simulink model "MHILSimHWImpl"  (R2024a)
settings: Solver=FixedStepDiscrete  StartTime=0.0  StopTime=2e-4  FixedStep=4e-9  RelTol=1e-3
values from neighbouring files (symbols this model uses):
  cfg = tddbl_model    [HILSimModel.m]
undefined symbols (not defined in the file or in its folder): AXI4, dt, hw, ip, Lite, xc7z020clg400
libraries: hdlBasic x1497, hdlUtilities x3, vmcUtilities x1
(part 3 of 11)

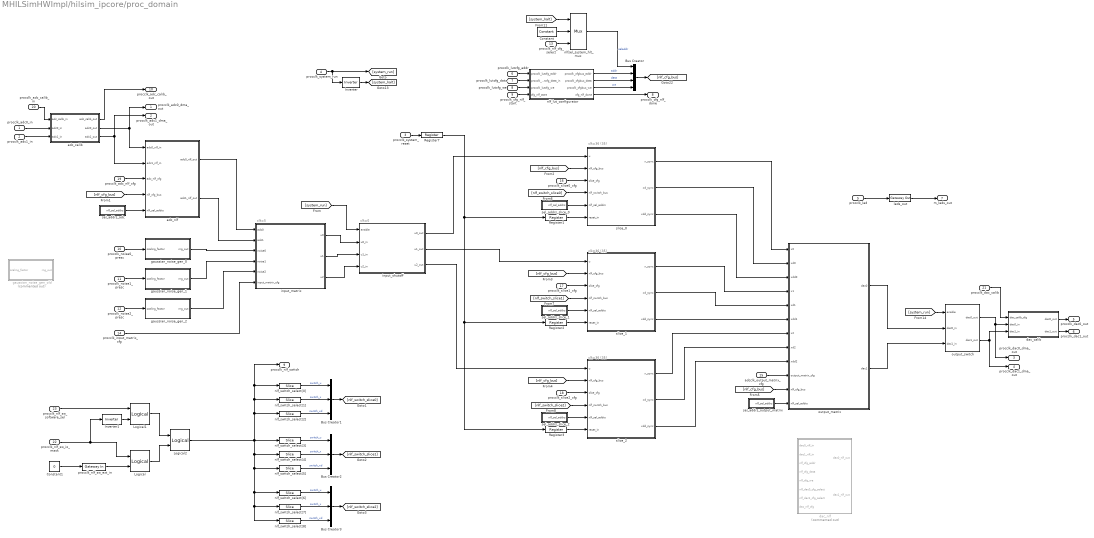
== system MHILSimHWImpl/hilsim_ipcore/proc_domain ==
  note: clk=5
  note: clk=0
  note: clk=36 (35)
  note: clk=36 (35)
  note: clk=36 (35)
  procclk_adc0_in : Inport
  procclk_adc1_in : Inport  Port=2
  procclk_system_reset : Inport  Port=3
  procclk_system_run : Inport  Port=4
  procclk_led : Inport  Port=5
  procclk_lutcfg_addr : Inport  Port=6
  procclk_lutcfg_data : Inport  Port=7
  procclk_lutcfg_we : Inport  Port=8
  procclk_cfg_nlf_start : Inport  Port=9
  procclk_noise0_presc : Inport  Port=10
  procclk_noise1_presc : Inport  Port=11
  procclk_noise2_presc : Inport  Port=12
  procclk_nlf_cfg_select : Inport  Port=13
  procclk_input_matrix_cfg : Inport  Port=14
  adcclk_output_matrix_cfg : Inport  Port=15
  procclk_slice0_cfg : Inport  Port=16
  procclk_slice1_cfg : Inport  Port=17
  procclk_slice2_cfg : Inport  Port=18
  procclk_adc_nlf_cfg : Inport  Port=19
  procclk_adc_calib_in : Inport  Port=20
  procclk_dac_calib : Inport  Port=21
  procclk_nlf_sw_io_mask : Inport  Port=22
  procclk_nlf_sw_software_sel : Inport  Port=23
  Bus Creator : BusCreator  Inputs=4
  Bus Creator1 : BusCreator  Inputs=3
  Bus Creator2 : BusCreator  Inputs=3
  Bus Creator3 : BusCreator  Inputs=3
  Constant : hdlBasic/Constant  const=255  gui_display_data_type=Fixed-point  arith_type=Unsigned  n_bits=8  bin_pt=0  preci_type=Single  exp_width=8  frac_width=24  explicit_period=off  period=1  XmcBlockStatus=1  maskContainerNames=tabcontainer1  block_type=constant  block_config=sysgen:Constant_config
  Constant1 : Constant  Value=0
  Inverter : hdlBasic/Inverter  en=off  latency=0  XmcBlockStatus=1  maskContainerNames=group2  block_type=inv  block_config=sysgen:Inverter_config
  Inverter1 : hdlBasic/Inverter  en=off  latency=0  XmcBlockStatus=1  maskContainerNames=group2  block_type=inv  block_config=sysgen:Inverter_config
  Logical : hdlBasic/Logical  logical_function=AND  inputs=2  en=off  latency=1  precision=Full  arith_type=Unsigned  n_bits=16  bin_pt=0  align_bp=on  overflow=[]  quantization=[]  XmcBlockStatus=1  maskContainerNames=tabcontainer1  block_type=logical  block_config=sysgen:Logical_config
  Logical1 : hdlBasic/Logical  logical_function=AND  inputs=2  en=off  latency=1  precision=Full  arith_type=Unsigned  n_bits=16  bin_pt=0  align_bp=on  overflow=[]  quantization=[]  XmcBlockStatus=1  maskContainerNames=tabcontainer1  block_type=logical  block_config=sysgen:Logical_config
  Logical2 : hdlBasic/Logical  logical_function=OR  inputs=2  en=off  latency=0  precision=Full  arith_type=Unsigned  n_bits=16  bin_pt=0  align_bp=on  overflow=[]  quantization=[]  XmcBlockStatus=1  maskContainerNames=tabcontainer1  block_type=logical  block_config=sysgen:Logical_config
  Register{1..3,7} (4 alike) : hdlBasic/Register  init=0  rst=off  en=off  XmcBlockStatus=1  maskContainerNames=tabcontainer1  block_type=register  block_config=sysgen:Register_config
  adc_calib : Subsystem
  adc_nlf : Subsystem
  dac_calib : Subsystem
  dac_nlf : Subsystem  Commented=on
  gaussian_noise_gen_0 : Subsystem
  gaussian_noise_gen_1 : Subsystem
  gaussian_noise_gen_2 : Subsystem
  gaussian_noise_gen_old : Subsystem  Commented=on
  input_matrix : Subsystem
  input_shutoff : Subsystem
  leds_out : hdlBasic/Gateway Out  inherit_from_input=off  hdl_port=on  rows=1  columns=1  UseAsDAC=off  DACChannel='1'  interface=None  automatic_assignment=on  address_offset=hex2dec('00')  intf_name=''  intf_description=''  timing_constraint=None  locs_specified=off  LOCs={}  io_standard={}  XmcBlockStatus=1  maskContainerNames=group4  block_type=gatewayout  block_config=sysgen:gateway_out_config  block_width_w=590  block_height_w=620  block_width=620  block_height=750
  nlf_lut_configurator : Subsystem
  nlf_switch_select[0] : hdlBasic/Slice  nbits=0  boolean_output=on  mode=Lower Bit Location + Width  bit1=0  base1=MSB of Input  bit0=0  base0=LSB of Input  XmcBlockStatus=1  maskContainerNames=group1  block_type=slice  block_config=sysgen:Slice_config
  nlf_switch_select[1] : hdlBasic/Slice  nbits=0  boolean_output=on  mode=Lower Bit Location + Width  bit1=0  base1=MSB of Input  bit0=1  base0=LSB of Input  XmcBlockStatus=1  maskContainerNames=group1  block_type=slice  block_config=sysgen:Slice_config
  nlf_switch_select[2] : hdlBasic/Slice  nbits=0  boolean_output=on  mode=Lower Bit Location + Width  bit1=0  base1=MSB of Input  bit0=2  base0=LSB of Input  XmcBlockStatus=1  maskContainerNames=group1  block_type=slice  block_config=sysgen:Slice_config
  nlf_switch_select[3] : hdlBasic/Slice  nbits=0  boolean_output=on  mode=Lower Bit Location + Width  bit1=0  base1=MSB of Input  bit0=3  base0=LSB of Input  XmcBlockStatus=1  maskContainerNames=group1  block_type=slice  block_config=sysgen:Slice_config
  nlf_switch_select[4] : hdlBasic/Slice  nbits=0  boolean_output=on  mode=Lower Bit Location + Width  bit1=0  base1=MSB of Input  bit0=4  base0=LSB of Input  XmcBlockStatus=1  maskContainerNames=group1  block_type=slice  block_config=sysgen:Slice_config
  nlf_switch_select[5] : hdlBasic/Slice  nbits=0  boolean_output=on  mode=Lower Bit Location + Width  bit1=0  base1=MSB of Input  bit0=5  base0=LSB of Input  XmcBlockStatus=1  maskContainerNames=group1  block_type=slice  block_config=sysgen:Slice_config
  nlf_switch_select[6] : hdlBasic/Slice  nbits=0  boolean_output=on  mode=Lower Bit Location + Width  bit1=0  base1=MSB of Input  bit0=6  base0=LSB of Input  XmcBlockStatus=1  maskContainerNames=group1  block_type=slice  block_config=sysgen:Slice_config
  nlf_switch_select[7] : hdlBasic/Slice  nbits=0  boolean_output=on  mode=Lower Bit Location + Width  bit1=0  base1=MSB of Input  bit0=7  base0=LSB of Input  XmcBlockStatus=1  maskContainerNames=group1  block_type=slice  block_config=sysgen:Slice_config
  nlf_switch_select[8] : hdlBasic/Slice  nbits=0  boolean_output=on  mode=Lower Bit Location + Width  bit1=0  base1=MSB of Input  bit0=8  base0=LSB of Input  XmcBlockStatus=1  maskContainerNames=group1  block_type=slice  block_config=sysgen:Slice_config
  nlfsel_system_hlt_mux : hdlBasic/Mux  inputs=2  en=off  latency=1  precision=Full  arith_type=Unsigned  n_bits=16  bin_pt=14  quantization=Truncate  overflow=Wrap  XmcBlockStatus=1  maskContainerNames=tabcontainer1  block_type=mux  block_config=sysgen:Mux_config
  output_matrix : Subsystem
  output_switch : Subsystem
  procclk_nlf_sw_ext_in : hdlBasic/Gateway In  gui_display_data_type=Fixed-point  arith_type=Unsigned  n_bits=9  bin_pt=0  preci_type=Single  exp_width=8  frac_width=24  rows=1  columns=1  quantization="Round  (unbiased: +/- Inf)"  overflow=Saturate  period=1  UseAsADC=off  ADCChannel='1'  interface=None  automatic_assignment=on  address_offset=hex2dec('00')  intf_name=''  intf_description=''  default_value=0  timing_constraint=None  locs_specified=off  LOCs={}  io_standard={}  inherit_from_input=off  hdl_port=on  XmcBlockStatus=1  maskContainerNames=group4  block_type=gatewayin  block_config=sysgen:gateway_in_config  block_width_w=590  block_height_w=620  block_width=640  block_height=850
  sel_addrs_adc : Subsystem
  sel_addrs_output_matrix : Subsystem
  sel_addrs_slice_0 : Subsystem
  sel_addrs_slice_1 : Subsystem
  sel_addrs_slice_2 : Subsystem
  slice_0 : Subsystem
  slice_1 : Subsystem
  slice_2 : Subsystem
  procclk_adc0_dma_out : Outport
  procclk_adc1_dma_out : Outport  Port=2
  procclk_dac0_dma_out : Outport  Port=3
  procclk_dac1_dma_out : Outport  Port=4
  procclk_dac0_out : Outport  Port=5
  procclk_dac1_out : Outport  Port=6
  m_leds_out : Outport  Port=7
  procclk_cfg_nlf_done : Outport  Port=8
  procclk_nlf_switch : Outport  Port=9
  procclk_adc_calib_out : Outport  Port=10
  wires:
  leds_out/1 -> m_leds_out/1
  procclk_led/1 -> leds_out/1
  procclk_lutcfg_addr/1 -> nlf_lut_configurator/1(procclk_lutcfg_addr)
  procclk_lutcfg_we/1 -> nlf_lut_configurator/3(procclk_lutcfg_we)
  procclk_lutcfg_data/1 -> nlf_lut_configurator/2(procclk_lutcfg_data_in)
  procclk_cfg_nlf_start/1 -> nlf_lut_configurator/4(cfg_nlf_start)
  nlf_lut_configurator/4(cfg_nlf_done) -> procclk_cfg_nlf_done/1
  procclk_slice0_cfg/1 -> slice_0/3(slice_cfg)
  gaussian_noise_gen_1/1(rng_out) -> input_matrix/4(noise1)
  gaussian_noise_gen_2/1(rng_out) -> input_matrix/5(noise2)
  procclk_noise0_presc/1 -> gaussian_noise_gen_0/1(scaling_factor)
  procclk_noise2_presc/1 -> gaussian_noise_gen_2/1(scaling_factor)
  procclk_noise1_presc/1 -> gaussian_noise_gen_1/1(scaling_factor)
  procclk_input_matrix_cfg/1 -> input_matrix/6(input_matrix_cfg)
  input_matrix/1(u0) -> input_shutoff/2(u0_in)
  input_matrix/2(u1) -> input_shutoff/3(u1_in)
  input_matrix/3(u2) -> input_shutoff/4(u2_in)
  [system_run] -> input_shutoff/1(enable)
  nlf_lut_configurator/1(procclk_cfgbus_addr) -> Bus Creator/2  "addr"
  nlf_lut_configurator/2(procclk_cfgbus_data) -> Bus Creator/3  "data"
  nlf_lut_configurator/3(procclk_cfgbus_we) -> Bus Creator/4  "we"
  input_shutoff/1(u0_out) -> slice_0/1(u)
  input_shutoff/2(u1_out) -> slice_1/1(u)
  input_shutoff/3(u2_out) -> slice_2/1(u)
  slice_0/1(x_sync) -> output_matrix/1(x0)
  slice_0/2(xd_sync) -> output_matrix/2(xd0)
  slice_1/1(x_sync) -> output_matrix/4(x1)
  slice_1/2(xd_sync) -> output_matrix/5(xd1)
  slice_2/1(x_sync) -> output_matrix/7(x2)
  slice_2/2(xd_sync) -> output_matrix/8(xd2)
  [system_run] -> output_switch/1(enable)
  adcclk_output_matrix_cfg/1 -> output_matrix/10(output_matrix_cfg)
  procclk_system_run/1 -> [system_run], Inverter/1
  Inverter/1 -> [system_halt]
  adc_nlf/2(adc1_nlf_out) -> input_matrix/2(adc1)
  adc_nlf/1(adc0_nlf_out) -> input_matrix/1(adc0)
  procclk_adc_nlf_cfg/1 -> adc_nlf/3(adc_nlf_cfg)
  gaussian_noise_gen_0/1(rng_out) -> input_matrix/3(noise0)
  procclk_system_reset/1 -> Register7/1
  Register7/1 -> Register3/1, Register2/1, Register1/1
  Register1/1 -> slice_0/6(reset_in)
  procclk_adc0_in/1 -> adc_calib/2(adc0_in)
  procclk_adc1_in/1 -> adc_calib/3(adc1_in)
  adc_calib/1(adc_calib_out) -> procclk_adc_calib_out/1
  procclk_adc_calib_in/1 -> adc_calib/1(adc_calib_in)
  adc_calib/2(adc0_out) -> procclk_adc0_dma_out/1, adc_nlf/1(adc0_nlf_in)
  adc_calib/3(adc1_out) -> procclk_adc1_dma_out/1, adc_nlf/2(adc1_nlf_in)
  output_matrix/1(dac0) -> output_switch/2(dac0_in)
  output_matrix/2(dac1) -> output_switch/3(dac1_in)
  dac_calib/1(dac0_out) -> procclk_dac0_out/1
  dac_calib/2(dac1_out) -> procclk_dac1_out/1
  output_switch/1(dac0_out) -> procclk_dac0_dma_out/1, dac_calib/2(dac0_in)
  output_switch/2(dac1_out) -> dac_calib/3(dac1_in), procclk_dac1_dma_out/1
  procclk_dac_calib/1 -> dac_calib/1(dac_calib_cfg)
  slice_0/3(xdd_sync) -> output_matrix/3(xdd0)
  slice_1/3(xdd_sync) -> output_matrix/6(xdd1)
  slice_2/3(xdd_sync) -> output_matrix/9(xdd2)
  Bus Creator/1 -> [nlf_cfg_bus]
  [nlf_cfg_bus] -> slice_0/2(nlf_cfg_bus)
  sel_addrs_slice_0/1(nlf_sel_addrs) -> slice_0/5(nlf_sel_addrs)
  [system_halt] -> nlfsel_system_hlt_mux/1
  nlfsel_system_hlt_mux/1 -> Bus Creator/1  "seladdr"
  procclk_slice1_cfg/1 -> slice_1/3(slice_cfg)
  Register2/1 -> slice_1/6(reset_in)
  sel_addrs_slice_1/1(nlf_sel_addrs) -> slice_1/5(nlf_sel_addrs)
  procclk_slice2_cfg/1 -> slice_2/3(slice_cfg)
  Register3/1 -> slice_2/6(reset_in)
  sel_addrs_slice_2/1(nlf_sel_addrs) -> slice_2/5(nlf_sel_addrs)
  sel_addrs_output_matrix/1(nlf_sel_addrs) -> output_matrix/12(nlf_sel_addrs)
  [nlf_cfg_bus] -> slice_1/2(nlf_cfg_bus)
  [nlf_cfg_bus] -> slice_2/2(nlf_cfg_bus)
  [nlf_cfg_bus] -> output_matrix/11(nlf_cfg_bus)
  sel_addrs_adc/1(nlf_sel_addrs) -> adc_nlf/5(nlf_sel_addrs)
  [nlf_cfg_bus] -> adc_nlf/4(nlf_cfg_bus)
  nlf_switch_select[0]/1 -> Bus Creator1/1  "switch_u"
  nlf_switch_select[1]/1 -> Bus Creator1/2  "switch_x"
  nlf_switch_select[2]/1 -> Bus Creator1/3  "switch_xd"
  Bus Creator1/1 -> [nlf_switch_slice0]
  [nlf_switch_slice0] -> slice_0/4(nlf_switch_bus)
  Bus Creator2/1 -> [nlf_switch_slice1]
  nlf_switch_select[5]/1 -> Bus Creator2/3  "switch_xd"
  nlf_switch_select[3]/1 -> Bus Creator2/1  "switch_u"
  nlf_switch_select[4]/1 -> Bus Creator2/2  "switch_x"
  [nlf_switch_slice1] -> slice_1/4(nlf_switch_bus)
  nlf_switch_select[6]/1 -> Bus Creator3/1  "switch_u"
  nlf_switch_select[8]/1 -> Bus Creator3/3  "switch_xd"
  nlf_switch_select[7]/1 -> Bus Creator3/2  "switch_x"
  Bus Creator3/1 -> [nlf_switch_slice2]
  [nlf_switch_slice2] -> slice_2/4(nlf_switch_bus)
  Logical2/1 -> procclk_nlf_switch/1, nlf_switch_select[0]/1, nlf_switch_select[1]/1, nlf_switch_select[2]/1, nlf_switch_select[8]/1, nlf_switch_select[7]/1, nlf_switch_select[6]/1, nlf_switch_select[5]/1, nlf_switch_select[4]/1, nlf_switch_select[3]/1
  Constant1/1 -> procclk_nlf_sw_ext_in/1
  procclk_nlf_sw_ext_in/1 -> Logical/2
  Inverter1/1 -> Logical1/2
  procclk_nlf_sw_io_mask/1 -> Inverter1/1, Logical/1
  procclk_nlf_sw_software_sel/1 -> Logical1/1
  Logical1/1 -> Logical2/1
  Logical/1 -> Logical2/2
  Constant/1 -> nlfsel_system_hlt_mux/2
  procclk_nlf_cfg_select/1 -> nlfsel_system_hlt_mux/3

== system MHILSimHWImpl/hilsim_ipcore/proc_domain/adc_calib ==
  adc_calib_in : Inport
  adc0_in : Inport  Port=2
  adc1_in : Inport  Port=3
  Bus Creator8 : BusCreator  Inputs=2
  Bus Selector9 : BusSelector  OutputSignals=signal1,signal2,signal3,signal4
  Register{1..3,17} (4 alike) : hdlBasic/Register  init=0  rst=off  en=off  XmcBlockStatus=1  maskContainerNames=tabcontainer1  block_type=register  block_config=sysgen:Register_config
  adc0_calib_add : hdlBasic/AddSub  mode=Addition  use_carryin=off  use_carryout=off  en=off  latency=1  precision=User Defined  arith_type="Signed  (2's comp)"  n_bits=dt.slice.sz  bin_pt=dt.slice.bin  quantization=Truncate  overflow=Wrap  use_behavioral_HDL=off  hw_selection=Fabric  pipelined=off  XmcBlockStatus=1  maskContainerNames=tabcontainer1  block_type=addsub  block_config=sysgen:Addsub_config
  adc0_calib_mul : hdlBasic/Mult  precision=User Defined  arith_type="Signed  (2's comp)"  n_bits=dt.slice.sz  bin_pt=dt.slice.bin  quantization=Truncate  overflow=Wrap  en=off  latency=3  opt_float=off  fp_mult_usage=No Usage  use_behavioral_HDL=off  opt=Speed  use_embedded=on  optimum_pipeline=off  pipeline=on  use_rpm=on  placement_style=Triangular  XmcBlockStatus=1  maskContainerNames=group1  block_type=mult  block_config=sysgen:Mult_config  block_width=598  block_height=876
  adc1_calib_add : hdlBasic/AddSub  mode=Addition  use_carryin=off  use_carryout=off  en=off  latency=1  precision=User Defined  arith_type="Signed  (2's comp)"  n_bits=dt.slice.sz  bin_pt=dt.slice.bin  quantization=Truncate  overflow=Wrap  use_behavioral_HDL=off  hw_selection=Fabric  pipelined=off  XmcBlockStatus=1  maskContainerNames=tabcontainer1  block_type=addsub  block_config=sysgen:Addsub_config
  adc1_calib_mul : hdlBasic/Mult  precision=User Defined  arith_type="Signed  (2's comp)"  n_bits=dt.slice.sz  bin_pt=dt.slice.bin  quantization=Truncate  overflow=Wrap  en=off  latency=3  opt_float=off  fp_mult_usage=No Usage  use_behavioral_HDL=off  opt=Speed  use_embedded=on  optimum_pipeline=off  pipeline=on  use_rpm=on  placement_style=Triangular  XmcBlockStatus=1  maskContainerNames=group1  block_type=mult  block_config=sysgen:Mult_config  block_width=598  block_height=876
  adc_calib_out : Outport
  adc0_out : Outport  Port=2
  adc1_out : Outport  Port=3
  wires:
  Bus Creator8/1 -> adc_calib_out/1
  adc0_in/1 -> adc0_calib_add/1
  adc0_calib_mul/1 -> Bus Creator8/1, adc0_out/1
  adc1_calib_mul/1 -> Bus Creator8/2, adc1_out/1
  adc1_in/1 -> adc1_calib_add/1
  Bus Selector9/2 -> Register1/1  "<signal2>"
  Bus Selector9/1 -> Register17/1  "<signal1>"
  adc0_calib_add/1 -> adc0_calib_mul/1
  adc1_calib_add/1 -> adc1_calib_mul/1
  Bus Selector9/3 -> Register2/1  "<signal3>"
  Bus Selector9/4 -> Register3/1  "<signal4>"
  adc_calib_in/1 -> Bus Selector9/1
  Register17/1 -> adc0_calib_add/2
  Register1/1 -> adc1_calib_add/2
  Register2/1 -> adc0_calib_mul/2
  Register3/1 -> adc1_calib_mul/2

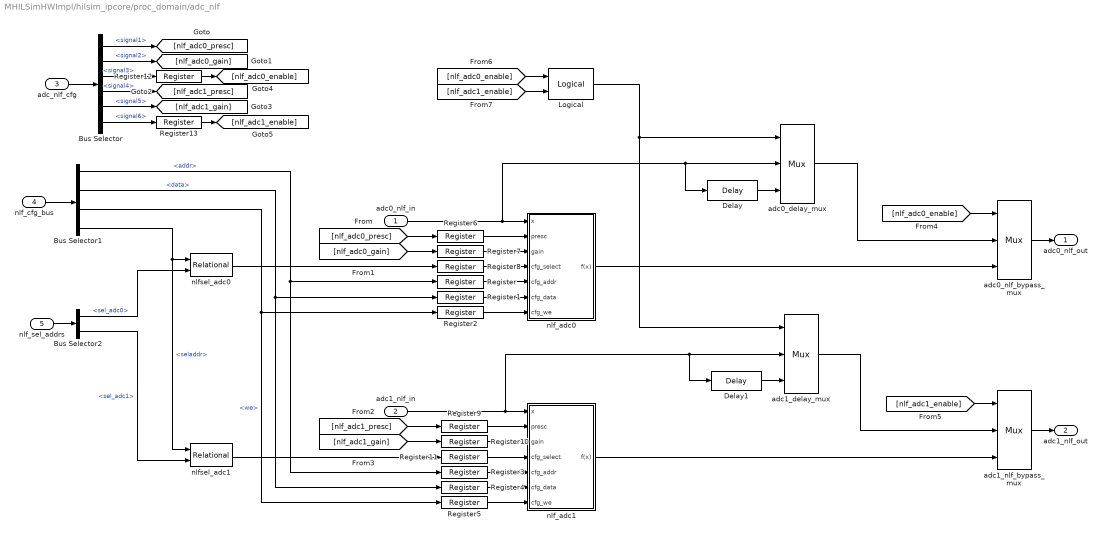
== system MHILSimHWImpl/hilsim_ipcore/proc_domain/adc_nlf ==
  adc0_nlf_in : Inport
  adc1_nlf_in : Inport  Port=2
  adc_nlf_cfg : Inport  Port=3
  nlf_cfg_bus : Inport  Port=4
  nlf_sel_addrs : Inport  Port=5
  Bus Selector : BusSelector  OutputSignals=signal1,signal2,signal3,signal4,signal5,signal6
  Bus Selector1 : BusSelector  OutputSignals=addr,data,we,seladdr
  Bus Selector2 : BusSelector  OutputSignals=sel_adc0,sel_adc1
  Delay : hdlBasic/Delay  rst=off  en=off  latency=12  reg_retiming=off  XmcBlockStatus=1  maskContainerNames=group1  block_type=delay  block_config=sysgen:Delay_config
  Delay1 : hdlBasic/Delay  rst=off  en=off  latency=12  reg_retiming=off  XmcBlockStatus=1  maskContainerNames=group1  block_type=delay  block_config=sysgen:Delay_config
  Logical : hdlBasic/Logical  logical_function=OR  inputs=2  en=off  latency=0  precision=Full  arith_type=Unsigned  n_bits=16  bin_pt=0  align_bp=on  overflow=[]  quantization=[]  XmcBlockStatus=1  maskContainerNames=tabcontainer1  block_type=logical  block_config=sysgen:Logical_config
  Register{,1..13} (14 alike) : hdlBasic/Register  init=0  rst=off  en=off  XmcBlockStatus=1  maskContainerNames=tabcontainer1  block_type=register  block_config=sysgen:Register_config
  adc0_delay_mux : hdlBasic/Mux  inputs=2  en=off  latency=0  precision=Full  arith_type=Unsigned  n_bits=16  bin_pt=14  quantization=Truncate  overflow=Wrap  XmcBlockStatus=1  maskContainerNames=tabcontainer1  block_type=mux  block_config=sysgen:Mux_config
  adc0_nlf_bypass_mux : hdlBasic/Mux  inputs=2  en=off  latency=1  precision=Full  arith_type=Unsigned  n_bits=16  bin_pt=14  quantization=Truncate  overflow=Wrap  XmcBlockStatus=1  maskContainerNames=tabcontainer1  block_type=mux  block_config=sysgen:Mux_config
  adc1_delay_mux : hdlBasic/Mux  inputs=2  en=off  latency=0  precision=Full  arith_type=Unsigned  n_bits=16  bin_pt=14  quantization=Truncate  overflow=Wrap  XmcBlockStatus=1  maskContainerNames=tabcontainer1  block_type=mux  block_config=sysgen:Mux_config
  adc1_nlf_bypass_mux : hdlBasic/Mux  inputs=2  en=off  latency=1  precision=Full  arith_type=Unsigned  n_bits=16  bin_pt=14  quantization=Truncate  overflow=Wrap  XmcBlockStatus=1  maskContainerNames=tabcontainer1  block_type=mux  block_config=sysgen:Mux_config
  nlf_adc0 : Subsystem
  nlf_adc1 : Subsystem
  nlfsel_adc0 : hdlBasic/Relational  mode=a=b  op_type=Bool  en=off  latency=1  XmcBlockStatus=1  maskContainerNames=tabcontainer1  block_type=relational  block_config=sysgen:Relational_config
  nlfsel_adc1 : hdlBasic/Relational  mode=a=b  op_type=Bool  en=off  latency=1  XmcBlockStatus=1  maskContainerNames=tabcontainer1  block_type=relational  block_config=sysgen:Relational_config
  adc0_nlf_out : Outport
  adc1_nlf_out : Outport  Port=2
  wires:
  adc0_nlf_in/1 -> nlf_adc0/1(x), Delay/1, adc0_delay_mux/2
  Register/1 -> nlf_adc0/5(cfg_addr)
  Register1/1 -> nlf_adc0/6(cfg_data)
  Register2/1 -> nlf_adc0/7(cfg_we)
  Register3/1 -> nlf_adc1/5(cfg_addr)
  Register5/1 -> nlf_adc1/7(cfg_we)
  Register4/1 -> nlf_adc1/6(cfg_data)
  Bus Selector1/1 -> Register/1, Register3/1  "<addr>"
  Bus Selector1/2 -> Register4/1, Register1/1  "<data>"
  Bus Selector1/3 -> Register5/1, Register2/1  "<we>"
  Register6/1 -> nlf_adc0/2(presc)
  Register7/1 -> nlf_adc0/3(gain)
  Register8/1 -> nlf_adc0/4(cfg_select)
  Register10/1 -> nlf_adc1/3(gain)
  Register9/1 -> nlf_adc1/2(presc)
  Register11/1 -> nlf_adc1/4(cfg_select)
  [nlf_adc0_presc] -> Register6/1
  [nlf_adc0_gain] -> Register7/1
  Bus Selector/1 -> [nlf_adc0_presc]  "<signal1>"
  Bus Selector/2 -> [nlf_adc0_gain]  "<signal2>"
  Bus Selector/3 -> Register12/1  "<signal3>"
  Bus Selector/4 -> [nlf_adc1_presc]  "<signal4>"
  [nlf_adc1_presc] -> Register9/1
  [nlf_adc1_gain] -> Register10/1
  adc0_nlf_bypass_mux/1 -> adc0_nlf_out/1
  nlf_adc0/1(f(x)) -> adc0_nlf_bypass_mux/3
  nlf_adc1/1(f(x)) -> adc1_nlf_bypass_mux/3
  adc1_nlf_bypass_mux/1 -> adc1_nlf_out/1
  [nlf_adc0_enable] -> adc0_nlf_bypass_mux/1
  [nlf_adc1_enable] -> adc1_nlf_bypass_mux/1
  Bus Selector/5 -> [nlf_adc1_gain]  "<signal5>"
  Bus Selector/6 -> Register13/1  "<signal6>"
  adc_nlf_cfg/1 -> Bus Selector/1
  [nlf_adc0_enable] -> Logical/1
  [nlf_adc1_enable] -> Logical/2
  Delay/1 -> adc0_delay_mux/3
  adc0_delay_mux/1 -> adc0_nlf_bypass_mux/2
  Delay1/1 -> adc1_delay_mux/3
  adc1_delay_mux/1 -> adc1_nlf_bypass_mux/2
  adc1_nlf_in/1 -> nlf_adc1/1(x), Delay1/1, adc1_delay_mux/2
  Logical/1 -> adc1_delay_mux/1, adc0_delay_mux/1
  Register12/1 -> [nlf_adc0_enable]
  Register13/1 -> [nlf_adc1_enable]
  nlf_cfg_bus/1 -> Bus Selector1/1
  nlfsel_adc0/1 -> Register8/1
  Bus Selector1/4 -> nlfsel_adc1/1, nlfsel_adc0/1  "<seladdr>"
  nlfsel_adc1/1 -> Register11/1
  nlf_sel_addrs/1 -> Bus Selector2/1
  Bus Selector2/1 -> nlfsel_adc0/2  "<sel_adc0>"
  Bus Selector2/2 -> nlfsel_adc1/2  "<sel_adc1>"

== system MHILSimHWImpl/hilsim_ipcore/proc_domain/dac_calib ==
  dac_calib_cfg : Inport
  dac0_in : Inport  Port=2
  dac1_in : Inport  Port=3
  Bus Selector : BusSelector  OutputSignals=signal1,signal2,signal3,signal4
  Register{1..4} (4 alike) : hdlBasic/Register  init=0  rst=off  en=off  XmcBlockStatus=1  maskContainerNames=tabcontainer1  block_type=register  block_config=sysgen:Register_config
  dac0_calib_add : hdlBasic/AddSub  mode=Addition  use_carryin=off  use_carryout=off  en=off  latency=1  precision=User Defined  arith_type="Signed  (2's comp)"  n_bits=dt.slice.sz  bin_pt=dt.slice.bin  quantization=Truncate  overflow=Wrap  use_behavioral_HDL=off  hw_selection=Fabric  pipelined=off  XmcBlockStatus=1  maskContainerNames=tabcontainer1  block_type=addsub  block_config=sysgen:Addsub_config
  dac0_calib_mul : hdlBasic/Mult  precision=User Defined  arith_type="Signed  (2's comp)"  n_bits=dt.slice.sz  bin_pt=dt.slice.bin  quantization=Truncate  overflow=Wrap  en=off  latency=3  opt_float=off  fp_mult_usage=No Usage  use_behavioral_HDL=off  opt=Speed  use_embedded=on  optimum_pipeline=off  pipeline=on  use_rpm=on  placement_style=Triangular  XmcBlockStatus=1  maskContainerNames=group1  block_type=mult  block_config=sysgen:Mult_config  block_width=598  block_height=876
  dac1_calib_add : hdlBasic/AddSub  mode=Addition  use_carryin=off  use_carryout=off  en=off  latency=1  precision=User Defined  arith_type="Signed  (2's comp)"  n_bits=dt.slice.sz  bin_pt=dt.slice.bin  quantization=Truncate  overflow=Wrap  use_behavioral_HDL=off  hw_selection=Fabric  pipelined=off  XmcBlockStatus=1  maskContainerNames=tabcontainer1  block_type=addsub  block_config=sysgen:Addsub_config
  dac1_calib_mul : hdlBasic/Mult  precision=User Defined  arith_type="Signed  (2's comp)"  n_bits=dt.slice.sz  bin_pt=dt.slice.bin  quantization=Truncate  overflow=Wrap  en=off  latency=3  opt_float=off  fp_mult_usage=No Usage  use_behavioral_HDL=off  opt=Speed  use_embedded=on  optimum_pipeline=off  pipeline=on  use_rpm=on  placement_style=Triangular  XmcBlockStatus=1  maskContainerNames=group1  block_type=mult  block_config=sysgen:Mult_config  block_width=598  block_height=876
  dac0_out : Outport
  dac1_out : Outport  Port=2
  wires:
  dac0_in/1 -> dac0_calib_mul/1
  dac0_calib_mul/1 -> dac0_calib_add/1
  dac0_calib_add/1 -> dac0_out/1
  dac1_calib_mul/1 -> dac1_calib_add/1
  dac1_calib_add/1 -> dac1_out/1
  dac1_in/1 -> dac1_calib_mul/1
  dac_calib_cfg/1 -> Bus Selector/1
  Bus Selector/1 -> Register3/1  "<signal1>"
  Bus Selector/2 -> Register2/1  "<signal2>"
  Bus Selector/3 -> Register1/1  "<signal3>"
  Bus Selector/4 -> Register4/1  "<signal4>"
  Register4/1 -> dac1_calib_mul/2
  Register1/1 -> dac0_calib_mul/2
  Register2/1 -> dac1_calib_add/2
  Register3/1 -> dac0_calib_add/2

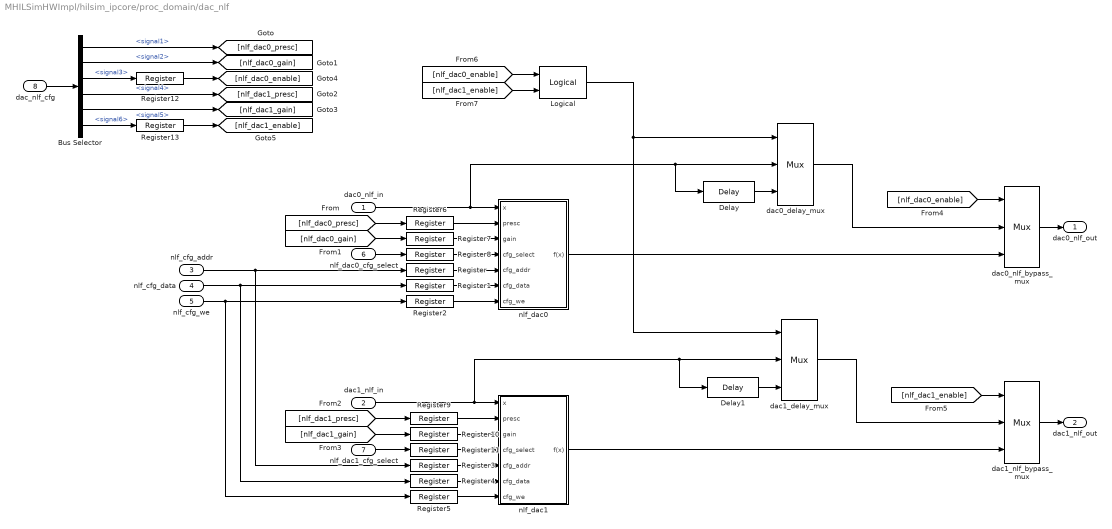
== system MHILSimHWImpl/hilsim_ipcore/proc_domain/dac_nlf ==
  dac0_nlf_in : Inport
  dac1_nlf_in : Inport  Port=2
  nlf_cfg_addr : Inport  Port=3
  nlf_cfg_data : Inport  Port=4
  nlf_cfg_we : Inport  Port=5
  nlf_dac0_cfg_select : Inport  Port=6
  nlf_dac1_cfg_select : Inport  Port=7
  dac_nlf_cfg : Inport  Port=8
  Bus Selector : BusSelector  OutputSignals=signal1,signal2,signal3,signal4,signal5,signal6
  Delay : hdlBasic/Delay  rst=off  en=off  latency=12  reg_retiming=off  XmcBlockStatus=1  maskContainerNames=group1  block_type=delay  block_config=sysgen:Delay_config
  Delay1 : hdlBasic/Delay  rst=off  en=off  latency=12  reg_retiming=off  XmcBlockStatus=1  maskContainerNames=group1  block_type=delay  block_config=sysgen:Delay_config
  Logical : hdlBasic/Logical  logical_function=OR  inputs=2  en=off  latency=0  precision=Full  arith_type=Unsigned  n_bits=16  bin_pt=0  align_bp=on  overflow=[]  quantization=[]  XmcBlockStatus=1  maskContainerNames=tabcontainer1  block_type=logical  block_config=sysgen:Logical_config
  Register{,1..13} (14 alike) : hdlBasic/Register  init=0  rst=off  en=off  XmcBlockStatus=1  maskContainerNames=tabcontainer1  block_type=register  block_config=sysgen:Register_config
  dac0_delay_mux : hdlBasic/Mux  inputs=2  en=off  latency=0  precision=Full  arith_type=Unsigned  n_bits=16  bin_pt=14  quantization=Truncate  overflow=Wrap  XmcBlockStatus=1  maskContainerNames=tabcontainer1  block_type=mux  block_config=sysgen:Mux_config
  dac0_nlf_bypass_mux : hdlBasic/Mux  inputs=2  en=off  latency=1  precision=Full  arith_type=Unsigned  n_bits=16  bin_pt=14  quantization=Truncate  overflow=Wrap  XmcBlockStatus=1  maskContainerNames=tabcontainer1  block_type=mux  block_config=sysgen:Mux_config
  dac1_delay_mux : hdlBasic/Mux  inputs=2  en=off  latency=0  precision=Full  arith_type=Unsigned  n_bits=16  bin_pt=14  quantization=Truncate  overflow=Wrap  XmcBlockStatus=1  maskContainerNames=tabcontainer1  block_type=mux  block_config=sysgen:Mux_config
  dac1_nlf_bypass_mux : hdlBasic/Mux  inputs=2  en=off  latency=1  precision=Full  arith_type=Unsigned  n_bits=16  bin_pt=14  quantization=Truncate  overflow=Wrap  XmcBlockStatus=1  maskContainerNames=tabcontainer1  block_type=mux  block_config=sysgen:Mux_config
  nlf_dac0 : Subsystem
  nlf_dac1 : Subsystem
  dac0_nlf_out : Outport
  dac1_nlf_out : Outport  Port=2
  wires:
  dac0_nlf_in/1 -> Delay/1, dac0_delay_mux/2, nlf_dac0/1(x)
  Register/1 -> nlf_dac0/5(cfg_addr)
  Register1/1 -> nlf_dac0/6(cfg_data)
  Register2/1 -> nlf_dac0/7(cfg_we)
  Register3/1 -> nlf_dac1/5(cfg_addr)
  Register5/1 -> nlf_dac1/7(cfg_we)
  Register4/1 -> nlf_dac1/6(cfg_data)
  nlf_cfg_addr/1 -> Register/1, Register3/1
  nlf_cfg_data/1 -> Register1/1, Register4/1
  nlf_cfg_we/1 -> Register2/1, Register5/1
  Register6/1 -> nlf_dac0/2(presc)
  Register7/1 -> nlf_dac0/3(gain)
  Register8/1 -> nlf_dac0/4(cfg_select)
  Register10/1 -> nlf_dac1/3(gain)
  Register9/1 -> nlf_dac1/2(presc)
  Register11/1 -> nlf_dac1/4(cfg_select)
  nlf_dac0_cfg_select/1 -> Register8/1
  nlf_dac1_cfg_select/1 -> Register11/1
  [nlf_dac0_presc] -> Register6/1
  [nlf_dac0_gain] -> Register7/1
  Bus Selector/1 -> [nlf_dac0_presc]  "<signal1>"
  Bus Selector/2 -> [nlf_dac0_gain]  "<signal2>"
  Bus Selector/3 -> Register12/1  "<signal3>"
  Bus Selector/4 -> [nlf_dac1_presc]  "<signal4>"
  [nlf_dac1_presc] -> Register9/1
  [nlf_dac1_gain] -> Register10/1
  dac0_nlf_bypass_mux/1 -> dac0_nlf_out/1
  nlf_dac0/1(f(x)) -> dac0_nlf_bypass_mux/3
  nlf_dac1/1(f(x)) -> dac1_nlf_bypass_mux/3
  dac1_nlf_bypass_mux/1 -> dac1_nlf_out/1
  [nlf_dac0_enable] -> dac0_nlf_bypass_mux/1
  [nlf_dac1_enable] -> dac1_nlf_bypass_mux/1
  Bus Selector/5 -> [nlf_dac1_gain]  "<signal5>"
  Bus Selector/6 -> Register13/1  "<signal6>"
  dac_nlf_cfg/1 -> Bus Selector/1
  dac0_delay_mux/1 -> dac0_nlf_bypass_mux/2
  Delay/1 -> dac0_delay_mux/3
  dac1_nlf_in/1 -> Delay1/1, dac1_delay_mux/2, nlf_dac1/1(x)
  dac1_delay_mux/1 -> dac1_nlf_bypass_mux/2
  Delay1/1 -> dac1_delay_mux/3
  Logical/1 -> dac1_delay_mux/1, dac0_delay_mux/1
  [nlf_dac0_enable] -> Logical/1
  [nlf_dac1_enable] -> Logical/2
  Register12/1 -> [nlf_dac0_enable]
  Register13/1 -> [nlf_dac1_enable]

== system MHILSimHWImpl/hilsim_ipcore/proc_domain/gaussian_noise_gen_0 ==
  note: LFSR constants:
      | lfsr_1: 0x927ce9
      | lfsr_2: 0x6c6d84
  scaling_factor : Inport
  Constant : hdlBasic/Constant  const=1.0  gui_display_data_type=Boolean  arith_type=Boolean  n_bits=16  bin_pt=14  preci_type=Single  exp_width=8  frac_width=24  explicit_period=on  period=hw.t_s*2  XmcBlockStatus=1  maskContainerNames=tabcontainer1  block_type=constant  block_config=sysgen:Constant_config
  Down Sample : hdlBasic/Down Sample  sample_ratio=hw.oversample/2  sample_phase="Last Value of Frame  (most efficient)"  en=off  rst=off  latency=1  XmcBlockStatus=1  maskContainerNames=group1  block_type=dsamp  block_config=sysgen:Downsample_config
  Down Sample1 : hdlBasic/Down Sample  sample_ratio=hw.oversample/2  sample_phase="Last Value of Frame  (most efficient)"  en=off  rst=off  latency=1  XmcBlockStatus=1  maskContainerNames=group1  block_type=dsamp  block_config=sysgen:Downsample_config
  Mult : hdlBasic/Mult  precision=User Defined  arith_type="Signed  (2's comp)"  n_bits=dt.slice.sz  bin_pt=dt.slice.bin  quantization=Truncate  overflow=Wrap  en=off  latency=3  opt_float=off  fp_mult_usage=No Usage  use_behavioral_HDL=off  opt=Speed  use_embedded=on  optimum_pipeline=off  pipeline=on  use_rpm=on  placement_style=Triangular  XmcBlockStatus=1  maskContainerNames=group1  block_type=mult  block_config=sysgen:Mult_config  block_width=598  block_height=876
  Up Sample : hdlBasic/Up Sample  sample_ratio=hw.oversample  copy_samples=on  en=off  latency=1  XmcBlockStatus=1  maskContainerNames=group1  block_type=usamp  block_config=sysgen:Upsample_config
  add_1_2 : hdlBasic/AddSub  mode=Addition  use_carryin=off  use_carryout=off  en=off  latency=1  precision=User Defined  arith_type="Signed  (2's comp)"  n_bits=13  bin_pt=7  quantization=Truncate  overflow=Wrap  use_behavioral_HDL=off  hw_selection=Fabric  pipelined=off  XmcBlockStatus=1  maskContainerNames=tabcontainer1  block_type=addsub  block_config=sysgen:Addsub_config
  lfsr_1 : hdlBasic/LFSR  lfsr_type=Galois  gate_type=XOR  n_bits=24  maxpolynomial=off  polynomial='c20001'  rst_value='927ce9'  rst=off  en=on  reloadable_seed=off  input_type=off  output_type=on  arith_type=Unsigned  bin_pt=0  explicit_period=off  period=1  XmcBlockStatus=1  maskContainerNames=tabcontainer1  block_type=lfsr  block_config=sysgen:LFSR_config
  lfsr_2 : hdlBasic/LFSR  lfsr_type=Galois  gate_type=XOR  n_bits=24  maxpolynomial=off  polynomial='c20001'  rst_value='6c6d84'  rst=off  en=on  reloadable_seed=off  input_type=off  output_type=on  arith_type=Unsigned  bin_pt=0  explicit_period=off  period=1  XmcBlockStatus=1  maskContainerNames=tabcontainer1  block_type=lfsr  block_config=sysgen:LFSR_config
  rom_box_muller_cos_1 : hdlBasic/ROM  depth=4096  initVector=ip.rng.box_muller_lut_cos  distributed_mem=Block RAM  rst=off  init_reg=0  en=off  latency=1  gui_display_data_type=Fixed-point  arith_type="Signed  (2's comp)"  n_bits=12  bin_pt=7  preci_type=Single  exp_width=8  frac_width=24  optimize=Area  use_rpm=on  simulation_type=fast_sim  XmcBlockStatus=1  maskContainerNames=tabcontainer1  block_type=sprom  block_config=sysgen:SPROM_config
  rom_box_muller_sin_1 : hdlBasic/ROM  depth=4096  initVector=ip.rng.box_muller_lut_sin  distributed_mem=Block RAM  rst=off  init_reg=0  en=off  latency=1  gui_display_data_type=Fixed-point  arith_type="Signed  (2's comp)"  n_bits=12  bin_pt=7  preci_type=Single  exp_width=8  frac_width=24  optimize=Area  use_rpm=on  simulation_type=fast_sim  XmcBlockStatus=1  maskContainerNames=tabcontainer1  block_type=sprom  block_config=sysgen:SPROM_config
  slice_1 : hdlBasic/Slice  nbits=12  boolean_output=off  mode=Lower Bit Location + Width  bit1=0  base1=MSB of Input  bit0=0  base0=LSB of Input  XmcBlockStatus=1  maskContainerNames=group1  block_type=slice  block_config=sysgen:Slice_config
  slice_2 : hdlBasic/Slice  nbits=12  boolean_output=off  mode=Lower Bit Location + Width  bit1=0  base1=MSB of Input  bit0=0  base0=LSB of Input  XmcBlockStatus=1  maskContainerNames=group1  block_type=slice  block_config=sysgen:Slice_config
  rng_out : Outport
  wires:
  add_1_2/1 -> Up Sample/1
  Mult/1 -> rng_out/1
  scaling_factor/1 -> Mult/2
  Up Sample/1 -> Mult/1
  Down Sample1/1 -> rom_box_muller_sin_1/1
  lfsr_1/1 -> slice_1/1
  Constant/1 -> lfsr_2/1, lfsr_1/1
  slice_1/1 -> Down Sample/1
  slice_2/1 -> Down Sample1/1
  Down Sample/1 -> rom_box_muller_cos_1/1
  rom_box_muller_sin_1/1 -> add_1_2/2
  rom_box_muller_cos_1/1 -> add_1_2/1
  lfsr_2/1 -> slice_2/1

== system MHILSimHWImpl/hilsim_ipcore/proc_domain/gaussian_noise_gen_1 ==
  note: LFSR constants:
      | lfsr_1: 0x18d035
      | lfsr_2: 0x30bc1c
  scaling_factor : Inport
  Constant : hdlBasic/Constant  const=1.0  gui_display_data_type=Boolean  arith_type=Boolean  n_bits=16  bin_pt=14  preci_type=Single  exp_width=8  frac_width=24  explicit_period=on  period=hw.t_s*2  XmcBlockStatus=1  maskContainerNames=tabcontainer1  block_type=constant  block_config=sysgen:Constant_config
  Down Sample : hdlBasic/Down Sample  sample_ratio=hw.oversample/2  sample_phase="Last Value of Frame  (most efficient)"  en=off  rst=off  latency=1  XmcBlockStatus=1  maskContainerNames=group1  block_type=dsamp  block_config=sysgen:Downsample_config
  Down Sample1 : hdlBasic/Down Sample  sample_ratio=hw.oversample/2  sample_phase="Last Value of Frame  (most efficient)"  en=off  rst=off  latency=1  XmcBlockStatus=1  maskContainerNames=group1  block_type=dsamp  block_config=sysgen:Downsample_config
  Mult : hdlBasic/Mult  precision=User Defined  arith_type="Signed  (2's comp)"  n_bits=dt.slice.sz  bin_pt=dt.slice.bin  quantization=Truncate  overflow=Wrap  en=off  latency=3  opt_float=off  fp_mult_usage=No Usage  use_behavioral_HDL=off  opt=Speed  use_embedded=on  optimum_pipeline=off  pipeline=on  use_rpm=on  placement_style=Triangular  XmcBlockStatus=1  maskContainerNames=group1  block_type=mult  block_config=sysgen:Mult_config  block_width=598  block_height=876
  Up Sample : hdlBasic/Up Sample  sample_ratio=hw.oversample  copy_samples=on  en=off  latency=1  XmcBlockStatus=1  maskContainerNames=group1  block_type=usamp  block_config=sysgen:Upsample_config
  add_1_2 : hdlBasic/AddSub  mode=Addition  use_carryin=off  use_carryout=off  en=off  latency=1  precision=User Defined  arith_type="Signed  (2's comp)"  n_bits=13  bin_pt=7  quantization=Truncate  overflow=Wrap  use_behavioral_HDL=off  hw_selection=Fabric  pipelined=off  XmcBlockStatus=1  maskContainerNames=tabcontainer1  block_type=addsub  block_config=sysgen:Addsub_config
  lfsr_1 : hdlBasic/LFSR  lfsr_type=Galois  gate_type=XOR  n_bits=24  maxpolynomial=off  polynomial='c20001'  rst_value='18d035'  rst=off  en=on  reloadable_seed=off  input_type=off  output_type=on  arith_type=Unsigned  bin_pt=0  explicit_period=off  period=1  XmcBlockStatus=1  maskContainerNames=tabcontainer1  block_type=lfsr  block_config=sysgen:LFSR_config
  lfsr_2 : hdlBasic/LFSR  lfsr_type=Galois  gate_type=XOR  n_bits=24  maxpolynomial=off  polynomial='c20001'  rst_value='30bc1c'  rst=off  en=on  reloadable_seed=off  input_type=off  output_type=on  arith_type=Unsigned  bin_pt=0  explicit_period=off  period=1  XmcBlockStatus=1  maskContainerNames=tabcontainer1  block_type=lfsr  block_config=sysgen:LFSR_config
  rom_box_muller_cos_1 : hdlBasic/ROM  depth=4096  initVector=ip.rng.box_muller_lut_cos  distributed_mem=Block RAM  rst=off  init_reg=0  en=off  latency=1  gui_display_data_type=Fixed-point  arith_type="Signed  (2's comp)"  n_bits=12  bin_pt=7  preci_type=Single  exp_width=8  frac_width=24  optimize=Area  use_rpm=on  simulation_type=fast_sim  XmcBlockStatus=1  maskContainerNames=tabcontainer1  block_type=sprom  block_config=sysgen:SPROM_config
  rom_box_muller_sin_1 : hdlBasic/ROM  depth=4096  initVector=ip.rng.box_muller_lut_sin  distributed_mem=Block RAM  rst=off  init_reg=0  en=off  latency=1  gui_display_data_type=Fixed-point  arith_type="Signed  (2's comp)"  n_bits=12  bin_pt=7  preci_type=Single  exp_width=8  frac_width=24  optimize=Area  use_rpm=on  simulation_type=fast_sim  XmcBlockStatus=1  maskContainerNames=tabcontainer1  block_type=sprom  block_config=sysgen:SPROM_config
  slice_1 : hdlBasic/Slice  nbits=12  boolean_output=off  mode=Lower Bit Location + Width  bit1=0  base1=MSB of Input  bit0=0  base0=LSB of Input  XmcBlockStatus=1  maskContainerNames=group1  block_type=slice  block_config=sysgen:Slice_config
  slice_2 : hdlBasic/Slice  nbits=12  boolean_output=off  mode=Lower Bit Location + Width  bit1=0  base1=MSB of Input  bit0=0  base0=LSB of Input  XmcBlockStatus=1  maskContainerNames=group1  block_type=slice  block_config=sysgen:Slice_config
  rng_out : Outport
  wires:
  add_1_2/1 -> Up Sample/1
  Mult/1 -> rng_out/1
  scaling_factor/1 -> Mult/2
  Up Sample/1 -> Mult/1
  Down Sample1/1 -> rom_box_muller_sin_1/1
  lfsr_1/1 -> slice_1/1
  Constant/1 -> lfsr_2/1, lfsr_1/1
  slice_1/1 -> Down Sample/1
  slice_2/1 -> Down Sample1/1
  Down Sample/1 -> rom_box_muller_cos_1/1
  rom_box_muller_sin_1/1 -> add_1_2/2
  rom_box_muller_cos_1/1 -> add_1_2/1
  lfsr_2/1 -> slice_2/1

== system MHILSimHWImpl/hilsim_ipcore/proc_domain/gaussian_noise_gen_2 ==
  note: LFSR constants:
      | lfsr_1: 0x667d82
      | lfsr_2: 0x8ad4e2
  scaling_factor : Inport
  Constant : hdlBasic/Constant  const=1.0  gui_display_data_type=Boolean  arith_type=Boolean  n_bits=16  bin_pt=14  preci_type=Single  exp_width=8  frac_width=24  explicit_period=on  period=hw.t_s*2  XmcBlockStatus=1  maskContainerNames=tabcontainer1  block_type=constant  block_config=sysgen:Constant_config
  Down Sample : hdlBasic/Down Sample  sample_ratio=hw.oversample/2  sample_phase="Last Value of Frame  (most efficient)"  en=off  rst=off  latency=1  XmcBlockStatus=1  maskContainerNames=group1  block_type=dsamp  block_config=sysgen:Downsample_config
  Down Sample1 : hdlBasic/Down Sample  sample_ratio=hw.oversample/2  sample_phase="Last Value of Frame  (most efficient)"  en=off  rst=off  latency=1  XmcBlockStatus=1  maskContainerNames=group1  block_type=dsamp  block_config=sysgen:Downsample_config
  Mult : hdlBasic/Mult  precision=User Defined  arith_type="Signed  (2's comp)"  n_bits=dt.slice.sz  bin_pt=dt.slice.bin  quantization=Truncate  overflow=Wrap  en=off  latency=3  opt_float=off  fp_mult_usage=No Usage  use_behavioral_HDL=off  opt=Speed  use_embedded=on  optimum_pipeline=off  pipeline=on  use_rpm=on  placement_style=Triangular  XmcBlockStatus=1  maskContainerNames=group1  block_type=mult  block_config=sysgen:Mult_config  block_width=598  block_height=876
  Up Sample : hdlBasic/Up Sample  sample_ratio=hw.oversample  copy_samples=on  en=off  latency=1  XmcBlockStatus=1  maskContainerNames=group1  block_type=usamp  block_config=sysgen:Upsample_config
  add_1_2 : hdlBasic/AddSub  mode=Addition  use_carryin=off  use_carryout=off  en=off  latency=1  precision=User Defined  arith_type="Signed  (2's comp)"  n_bits=13  bin_pt=7  quantization=Truncate  overflow=Wrap  use_behavioral_HDL=off  hw_selection=Fabric  pipelined=off  XmcBlockStatus=1  maskContainerNames=tabcontainer1  block_type=addsub  block_config=sysgen:Addsub_config
  lfsr_1 : hdlBasic/LFSR  lfsr_type=Galois  gate_type=XOR  n_bits=24  maxpolynomial=off  polynomial='c20001'  rst_value='667d82'  rst=off  en=on  reloadable_seed=off  input_type=off  output_type=on  arith_type=Unsigned  bin_pt=0  explicit_period=off  period=1  XmcBlockStatus=1  maskContainerNames=tabcontainer1  block_type=lfsr  block_config=sysgen:LFSR_config
  lfsr_2 : hdlBasic/LFSR  lfsr_type=Galois  gate_type=XOR  n_bits=24  maxpolynomial=off  polynomial='c20001'  rst_value='8ad4e2'  rst=off  en=on  reloadable_seed=off  input_type=off  output_type=on  arith_type=Unsigned  bin_pt=0  explicit_period=off  period=1  XmcBlockStatus=1  maskContainerNames=tabcontainer1  block_type=lfsr  block_config=sysgen:LFSR_config
  rom_box_muller_cos_1 : hdlBasic/ROM  depth=4096  initVector=ip.rng.box_muller_lut_cos  distributed_mem=Block RAM  rst=off  init_reg=0  en=off  latency=1  gui_display_data_type=Fixed-point  arith_type="Signed  (2's comp)"  n_bits=12  bin_pt=7  preci_type=Single  exp_width=8  frac_width=24  optimize=Area  use_rpm=on  simulation_type=fast_sim  XmcBlockStatus=1  maskContainerNames=tabcontainer1  block_type=sprom  block_config=sysgen:SPROM_config
  rom_box_muller_sin_1 : hdlBasic/ROM  depth=4096  initVector=ip.rng.box_muller_lut_sin  distributed_mem=Block RAM  rst=off  init_reg=0  en=off  latency=1  gui_display_data_type=Fixed-point  arith_type="Signed  (2's comp)"  n_bits=12  bin_pt=7  preci_type=Single  exp_width=8  frac_width=24  optimize=Area  use_rpm=on  simulation_type=fast_sim  XmcBlockStatus=1  maskContainerNames=tabcontainer1  block_type=sprom  block_config=sysgen:SPROM_config
  slice_1 : hdlBasic/Slice  nbits=12  boolean_output=off  mode=Lower Bit Location + Width  bit1=0  base1=MSB of Input  bit0=0  base0=LSB of Input  XmcBlockStatus=1  maskContainerNames=group1  block_type=slice  block_config=sysgen:Slice_config
  slice_2 : hdlBasic/Slice  nbits=12  boolean_output=off  mode=Lower Bit Location + Width  bit1=0  base1=MSB of Input  bit0=0  base0=LSB of Input  XmcBlockStatus=1  maskContainerNames=group1  block_type=slice  block_config=sysgen:Slice_config
  rng_out : Outport
  wires:
  add_1_2/1 -> Up Sample/1
  Mult/1 -> rng_out/1
  scaling_factor/1 -> Mult/2
  Up Sample/1 -> Mult/1
  Down Sample1/1 -> rom_box_muller_sin_1/1
  lfsr_1/1 -> slice_1/1
  Constant/1 -> lfsr_2/1, lfsr_1/1
  slice_1/1 -> Down Sample/1
  slice_2/1 -> Down Sample1/1
  Down Sample/1 -> rom_box_muller_cos_1/1
  rom_box_muller_sin_1/1 -> add_1_2/2
  rom_box_muller_cos_1/1 -> add_1_2/1
  lfsr_2/1 -> slice_2/1

== system MHILSimHWImpl/hilsim_ipcore/proc_domain/gaussian_noise_gen_old ==
  scaling_factor : Inport
  Constant : hdlBasic/Constant  const=1.0  gui_display_data_type=Boolean  arith_type=Boolean  n_bits=16  bin_pt=14  preci_type=Single  exp_width=8  frac_width=24  explicit_period=on  period=hw.t_s*hw.oversample  XmcBlockStatus=1  maskContainerNames=tabcontainer1  block_type=constant  block_config=sysgen:Constant_config
  Mult : hdlBasic/Mult  precision=User Defined  arith_type="Signed  (2's comp)"  n_bits=dt.slice.sz  bin_pt=dt.slice.bin  quantization=Truncate  overflow=Wrap  en=off  latency=3  use_behavioral_HDL=off  opt=Speed  use_embedded=on  optimum_pipeline=off  pipeline=on  use_rpm=on  placement_style=Triangular  XmcBlockStatus=1  maskContainerNames=group1  block_type=mult  block_config=sysgen:Mult_config  block_width=598  block_height=876
  Up Sample : hdlBasic/Up Sample  sample_ratio=hw.oversample  copy_samples=on  en=off  latency=1  XmcBlockStatus=1  maskContainerNames=group1  block_type=usamp  block_config=sysgen:Upsample_config
  add_1_2 : hdlBasic/AddSub  mode=Addition  use_carryin=off  use_carryout=off  en=off  latency=1  precision=User Defined  arith_type="Signed  (2's comp)"  n_bits=13  bin_pt=7  quantization=Truncate  overflow=Wrap  use_behavioral_HDL=off  hw_selection=Fabric  pipelined=off  XmcBlockStatus=1  maskContainerNames=tabcontainer1  block_type=addsub  block_config=sysgen:Addsub_config
  add_3_4 : hdlBasic/AddSub  mode=Addition  use_carryin=off  use_carryout=off  en=off  latency=1  precision=User Defined  arith_type="Signed  (2's comp)"  n_bits=13  bin_pt=7  quantization=Truncate  overflow=Wrap  use_behavioral_HDL=off  hw_selection=Fabric  pipelined=off  XmcBlockStatus=1  maskContainerNames=tabcontainer1  block_type=addsub  block_config=sysgen:Addsub_config
  add_total : hdlBasic/AddSub  mode=Addition  use_carryin=off  use_carryout=off  en=off  latency=1  precision=User Defined  arith_type="Signed  (2's comp)"  n_bits=14  bin_pt=7  quantization=Truncate  overflow=Wrap  use_behavioral_HDL=off  hw_selection=Fabric  pipelined=off  XmcBlockStatus=1  maskContainerNames=tabcontainer1  block_type=addsub  block_config=sysgen:Addsub_config
  lfsr_1 : hdlBasic/LFSR  lfsr_type=Fibonacci  gate_type=XNOR  n_bits=16  maxpolynomial=on  polynomial='6805'  rst_value='f00d'  rst=off  en=on  reloadable_seed=off  input_type=off  output_type=on  arith_type=Unsigned  bin_pt=0  explicit_period=off  period=1  XmcBlockStatus=1  maskContainerNames=tabcontainer1  block_type=lfsr  block_config=sysgen:LFSR_config
  lfsr_2 : hdlBasic/LFSR  lfsr_type=Fibonacci  gate_type=XNOR  n_bits=13  maxpolynomial=on  polynomial='0807'  rst_value='02e3'  rst=off  en=on  reloadable_seed=off  input_type=off  output_type=on  arith_type=Unsigned  bin_pt=0  explicit_period=off  period=1  XmcBlockStatus=1  maskContainerNames=tabcontainer1  block_type=lfsr  block_config=sysgen:LFSR_config
  lfsr_3 : hdlBasic/LFSR  lfsr_type=Fibonacci  gate_type=XNOR  n_bits=15  maxpolynomial=on  polynomial='3001'  rst_value='1337'  rst=off  en=on  reloadable_seed=off  input_type=off  output_type=on  arith_type=Unsigned  bin_pt=0  explicit_period=off  period=1  XmcBlockStatus=1  maskContainerNames=tabcontainer1  block_type=lfsr  block_config=sysgen:LFSR_config
  lfsr_4 : hdlBasic/LFSR  lfsr_type=Fibonacci  gate_type=XNOR  n_bits=17  maxpolynomial=on  polynomial='09001'  rst_value='babe'  rst=off  en=on  reloadable_seed=off  input_type=off  output_type=on  arith_type=Unsigned  bin_pt=0  explicit_period=off  period=1  XmcBlockStatus=1  maskContainerNames=tabcontainer1  block_type=lfsr  block_config=sysgen:LFSR_config
  rom_box_muller_cos_1 : hdlBasic/ROM  depth=4096  initVector=ip.rng.box_muller_lut_cos  distributed_mem=Block RAM  rst=off  init_reg=0  en=off  latency=1  gui_display_data_type=Fixed-point  arith_type="Signed  (2's comp)"  n_bits=12  bin_pt=7  preci_type=Single  exp_width=8  frac_width=24  optimize=Area  use_rpm=on  simulation_type=fast_sim  XmcBlockStatus=1  maskContainerNames=tabcontainer1  block_type=sprom  block_config=sysgen:SPROM_config
  rom_box_muller_cos_2 : hdlBasic/ROM  depth=4096  initVector=ip.rng.box_muller_lut_cos  distributed_mem=Block RAM  rst=off  init_reg=0  en=off  latency=1  gui_display_data_type=Fixed-point  arith_type="Signed  (2's comp)"  n_bits=12  bin_pt=7  preci_type=Single  exp_width=8  frac_width=24  optimize=Area  use_rpm=on  simulation_type=fast_sim  XmcBlockStatus=1  maskContainerNames=tabcontainer1  block_type=sprom  block_config=sysgen:SPROM_config
  rom_box_muller_sin_1 : hdlBasic/ROM  depth=4096  initVector=ip.rng.box_muller_lut_sin  distributed_mem=Block RAM  rst=off  init_reg=0  en=off  latency=1  gui_display_data_type=Fixed-point  arith_type="Signed  (2's comp)"  n_bits=12  bin_pt=7  preci_type=Single  exp_width=8  frac_width=24  optimize=Area  use_rpm=on  simulation_type=fast_sim  XmcBlockStatus=1  maskContainerNames=tabcontainer1  block_type=sprom  block_config=sysgen:SPROM_config
  rom_box_muller_sin_2 : hdlBasic/ROM  depth=4096  initVector=ip.rng.box_muller_lut_sin  distributed_mem=Block RAM  rst=off  init_reg=0  en=off  latency=1  gui_display_data_type=Fixed-point  arith_type="Signed  (2's comp)"  n_bits=12  bin_pt=7  preci_type=Single  exp_width=8  frac_width=24  optimize=Area  use_rpm=on  simulation_type=fast_sim  XmcBlockStatus=1  maskContainerNames=tabcontainer1  block_type=sprom  block_config=sysgen:SPROM_config
  slice_1 : hdlBasic/Slice  nbits=12  boolean_output=off  mode=Lower Bit Location + Width  bit1=0  base1=MSB of Input  bit0=0  base0=LSB of Input  XmcBlockStatus=1  maskContainerNames=group1  block_type=slice  block_config=sysgen:Slice_config
  slice_2 : hdlBasic/Slice  nbits=12  boolean_output=off  mode=Lower Bit Location + Width  bit1=0  base1=MSB of Input  bit0=0  base0=LSB of Input  XmcBlockStatus=1  maskContainerNames=group1  block_type=slice  block_config=sysgen:Slice_config
  slice_3 : hdlBasic/Slice  nbits=12  boolean_output=off  mode=Lower Bit Location + Width  bit1=0  base1=MSB of Input  bit0=1  base0=LSB of Input  XmcBlockStatus=1  maskContainerNames=group1  block_type=slice  block_config=sysgen:Slice_config
  slice_4 : hdlBasic/Slice  nbits=12  boolean_output=off  mode=Lower Bit Location + Width  bit1=0  base1=MSB of Input  bit0=3  base0=LSB of Input  XmcBlockStatus=1  maskContainerNames=group1  block_type=slice  block_config=sysgen:Slice_config
  rng_out : Outport
  wires:
  slice_1/1 -> rom_box_muller_cos_1/1
  lfsr_1/1 -> slice_1/1
  lfsr_2/1 -> slice_2/1
  slice_2/1 -> rom_box_muller_sin_1/1
  Constant/1 -> lfsr_4/1, lfsr_3/1, lfsr_2/1, lfsr_1/1
  lfsr_3/1 -> slice_3/1
  lfsr_4/1 -> slice_4/1
  slice_4/1 -> rom_box_muller_sin_2/1
  slice_3/1 -> rom_box_muller_cos_2/1
  rom_box_muller_cos_2/1 -> add_3_4/1
  rom_box_muller_sin_2/1 -> add_3_4/2
  rom_box_muller_sin_1/1 -> add_1_2/2
  rom_box_muller_cos_1/1 -> add_1_2/1
  add_1_2/1 -> add_total/1
  add_3_4/1 -> add_total/2
  add_total/1 -> Up Sample/1
  Mult/1 -> rng_out/1
  scaling_factor/1 -> Mult/2
  Up Sample/1 -> Mult/1
